simulink library "Over_Voltage_Protection_Relay"  (R2024a)
settings: Solver=VariableStepAuto  StartTime=0.0  StopTime=10.0  RelTol=1e-3
libraries: simulink_extras x3, spsThreePhaseVIMeasurementLib x1, spsThreePhaseBreakerLib x1
settings Model: Creator=gshma  LastModifiedBy=gshma

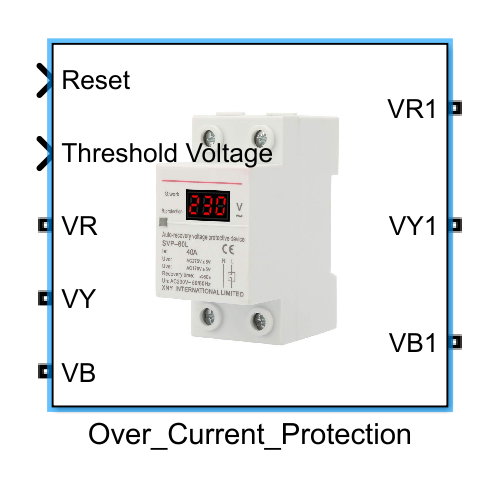
[thumbnail: Simulink's stored preview of the top-level diagram]
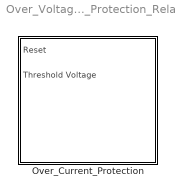
== system Over_Voltage_Protection_Relay ==
  Over_Current_Protection : Subsystem
      mask Display: image('over_voltage_prot_image.jpg', [0,0,0,0,75,75]);

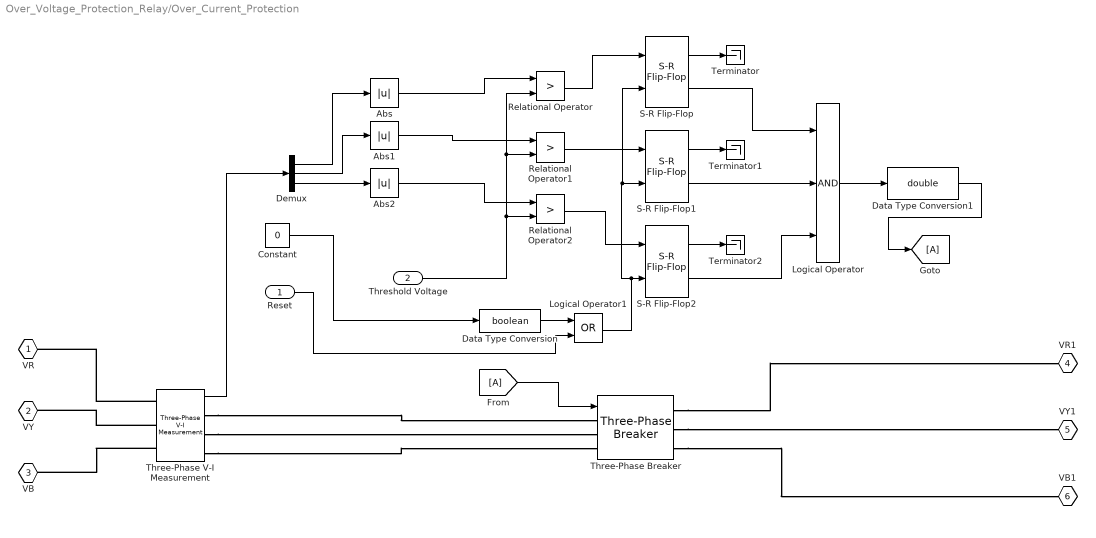
== system Over_Voltage_Protection_Relay/Over_Current_Protection ==
  Reset : Inport
  Threshold Voltage : Inport  Port=2
  Abs : Abs  SaturateOnIntegerOverflow=off
  Abs1 : Abs  SaturateOnIntegerOverflow=off
  Abs2 : Abs  SaturateOnIntegerOverflow=off
  Constant : Constant  Value=0  SampleTime=0.001
  Data Type Conversion : DataTypeConversion  OutDataTypeStr=boolean  SaturateOnIntegerOverflow=off  RndMeth=Floor
  Data Type Conversion1 : DataTypeConversion  OutDataTypeStr=double  SaturateOnIntegerOverflow=off  RndMeth=Floor
  Demux : Demux  Outputs=3
  From : From
  Goto : Goto
  Logical Operator : Logic  Inputs=3  AllPortsSameDT=off  OutDataTypeStr=boolean
  Logical Operator1 : Logic  Operator=OR  AllPortsSameDT=off  OutDataTypeStr=boolean
  Relational Operator : RelationalOperator  Operator=>  OutDataTypeStr=boolean  RndMeth=Simplest  InputSameDT=off
  Relational Operator1 : RelationalOperator  Operator=>  OutDataTypeStr=boolean  RndMeth=Simplest  InputSameDT=off
  Relational Operator2 : RelationalOperator  Operator=>  OutDataTypeStr=boolean  RndMeth=Simplest  InputSameDT=off
  S-R Flip-Flop : simulink_extras/Flip Flops/S-R Flip-Flop  initial_condition=0
  S-R Flip-Flop1 : simulink_extras/Flip Flops/S-R Flip-Flop  initial_condition=0
  S-R Flip-Flop2 : simulink_extras/Flip Flops/S-R Flip-Flop  initial_condition=0
  Terminator : Terminator
  Terminator1 : Terminator
  Terminator2 : Terminator
  Three-Phase V-I Measurement : spsThreePhaseVIMeasurementLib/Three-Phase V-I Measurement  VoltageMeasurement=phase-to-phase  SetLabelV=off  LabelV=Vabc  Vpu=off  VpuLL=off  CurrentMeasurement=no  SetLabelI=off  LabelI=Iabc  Ipu=off  Pbase=100e6  Vbase=500e3  OutputType=Complex  PhasorSimulation=off  PSBequivalent=0
  Three-Phase Breaker : spsThreePhaseBreakerLib/Three-Phase Breaker  InitialState=closed  SwitchA=on  SwitchB=on  SwitchC=on  SwitchTimes="[1/60  5/60]"  External=on  BreakerResistance=0.01  SnubberResistance=1e6  SnubberCapacitance=inf  Measurements=None
  VR : PMIOPort  Tag=simrfV2util1/Connection Port  Side=Left
  VY : PMIOPort  Tag=simrfV2util1/Connection Port  Port=2  Side=Left
  VB : PMIOPort  Tag=simrfV2util1/Connection Port  Port=3  Side=Left
  VR1 : PMIOPort  Tag=simrfV2util1/Connection Port  Port=4  Side=Right
  VY1 : PMIOPort  Tag=simrfV2util1/Connection Port  Port=5  Side=Right
  VB1 : PMIOPort  Tag=simrfV2util1/Connection Port  Port=6  Side=Right
  wires:
  Abs2/1 -> Relational Operator2/1
  Abs1/1 -> Relational Operator1/1
  Abs/1 -> Relational Operator/1
  Threshold Voltage/1 -> Relational Operator2/2, Relational Operator1/2, Relational Operator/2
  Relational Operator/1 -> S-R Flip-Flop/1
  Relational Operator1/1 -> S-R Flip-Flop1/1
  Relational Operator2/1 -> S-R Flip-Flop2/1
  Constant/1 -> Data Type Conversion/1
  Data Type Conversion/1 -> Logical Operator1/1
  S-R Flip-Flop/2 -> Logical Operator/1
  S-R Flip-Flop1/2 -> Logical Operator/2
  S-R Flip-Flop2/2 -> Logical Operator/3
  S-R Flip-Flop2/1 -> Terminator2/1
  S-R Flip-Flop1/1 -> Terminator1/1
  S-R Flip-Flop/1 -> Terminator/1
  From/1 -> Three-Phase Breaker/1
  Logical Operator/1 -> Data Type Conversion1/1
  Data Type Conversion1/1 -> Goto/1
  Three-Phase V-I Measurement/1 -> Demux/1
  Demux/1 -> Abs/1
  Demux/2 -> Abs1/1
  Demux/3 -> Abs2/1
  Reset/1 -> Logical Operator1/2
  Logical Operator1/1 -> S-R Flip-Flop1/2, S-R Flip-Flop/2, S-R Flip-Flop2/2
  connections:
  Three-Phase Breaker/RConn1 -- VR1/RConn1
  Three-Phase Breaker/RConn2 -- VY1/RConn1
  Three-Phase Breaker/RConn3 -- VB1/RConn1
  Three-Phase V-I Measurement/RConn1 -- Three-Phase Breaker/LConn1
  Three-Phase V-I Measurement/RConn2 -- Three-Phase Breaker/LConn2
  Three-Phase V-I Measurement/RConn3 -- Three-Phase Breaker/LConn3
  Three-Phase V-I Measurement/LConn1 -- VR/RConn1
  Three-Phase V-I Measurement/LConn2 -- VY/RConn1
  Three-Phase V-I Measurement/LConn3 -- VB/RConn1
